simulink model "LQG_sim_no_friction"  (R2024b)
settings: Solver=ode4  StartTime=0.0  StopTime=T  FixedStep=Ts  RelTol=1e-3
values from neighbouring files (symbols this model uses):
  D = [0 0]'    [IP_MACRO.m]
  K = lqr(A, B, Qr, Rr)    [IP_MACRO.m]
  L = lqe(A, G, C, Qe, Re)    [IP_MACRO.m]
  x0 = [0.1 1 0.2 0 0]'    [IP_MACRO.m]
undefined symbols (not defined in the file or in its folder): A, B, C, dead_zone, noise_power, noise_sample_time, saturation, tau
libraries: simulink x1
settings Model: Creator=leita  LastModifiedBy=leita
settings DataIOCC: ReturnWorkspaceOutputs=off

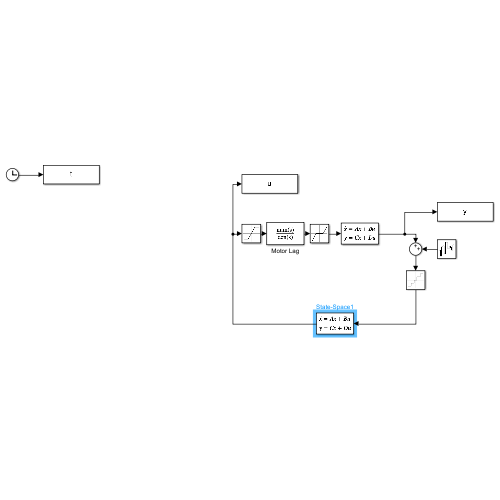
[thumbnail: Simulink's stored preview of the top-level diagram]
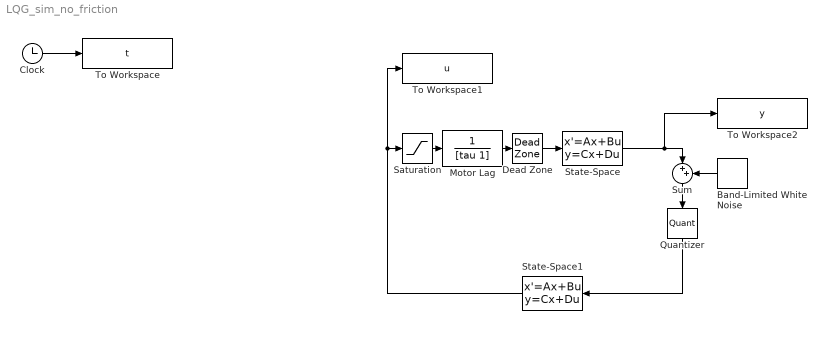
== system LQG_sim_no_friction ==
  Band-Limited White Noise : simulink/Sources/Band-Limited White Noise  Cov=[noise_power]  Ts=noise_sample_time  seed=[23341]
  Clock : Clock
  Dead Zone : DeadZone  LowerValue=-dead_zone  UpperValue=dead_zone
  Motor Lag : TransferFcn  Denominator=[tau 1]
  Quantizer : Quantizer  QuantizationInterval=quant
  Saturation : Saturate  UpperLimit=saturation  LowerLimit=-saturation
  State-Space : StateSpace  A=A  B=B  C=C  D=D  InitialCondition=x0
  State-Space1 : StateSpace  A=A-B*K-L*C  B=L  C=-K  D=D  InitialCondition=0
  Sum : Sum  Inputs=|++
  To Workspace : ToWorkspace  VariableName=t  SaveFormat=Timeseries  SampleTime=-1
  To Workspace1 : ToWorkspace  VariableName=u  SaveFormat=Timeseries  SampleTime=-1
  To Workspace2 : ToWorkspace  VariableName=y  SaveFormat=Timeseries  SampleTime=-1
  wires:
  State-Space1/1 -> To Workspace1/1, Saturation/1
  State-Space/1 -> To Workspace2/1, Sum/1
  Sum/1 -> Quantizer/1
  Quantizer/1 -> State-Space1/1
  Band-Limited White Noise/1 -> Sum/2
  Clock/1 -> To Workspace/1
  Saturation/1 -> Motor Lag/1
  Motor Lag/1 -> Dead Zone/1
  Dead Zone/1 -> State-Space/1
